simulink model "model2"  (R2025a)
settings: Solver=FixedStepAuto  StartTime=0.0  StopTime=3600  FixedStep=5  RelTol=1e-3
libraries: fuzblock x3
settings Model: Creator=boris  LastModifiedBy=boris

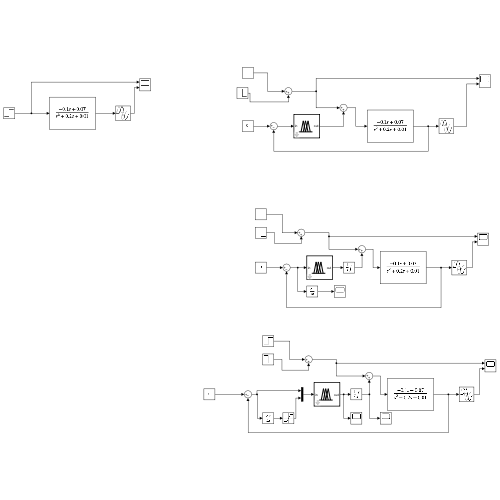
[thumbnail: Simulink's stored preview of the top-level diagram]
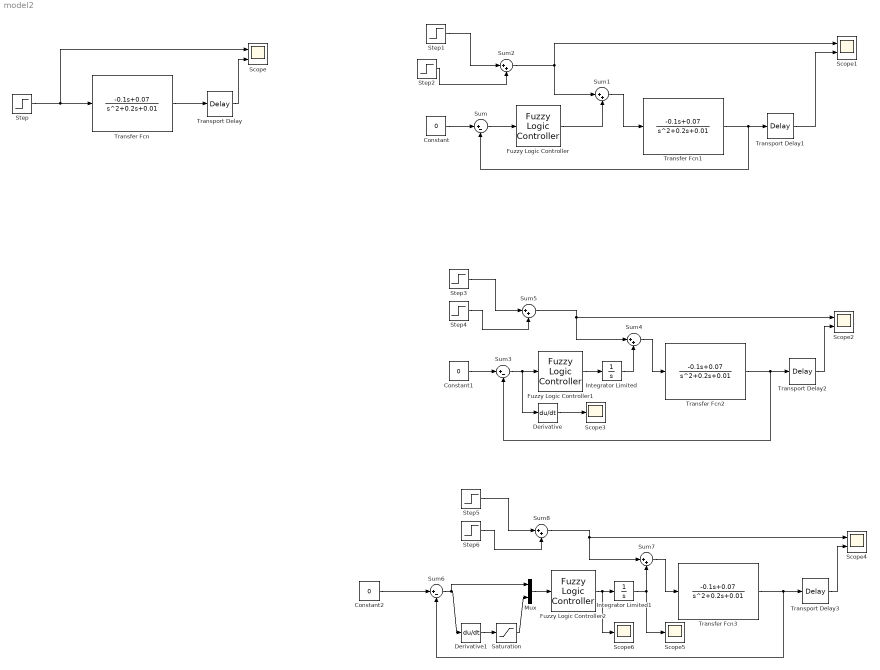
== system model2 ==
  Constant : Constant  Value=0
  Constant1 : Constant  Value=0
  Constant2 : Constant  Value=0
  Derivative : Derivative
  Derivative1 : Derivative
  Fuzzy Logic Controller : fuzblock/Fuzzy Logic  Controller  FIS='fisprvasema.fis'  OutputSampleNumber=101  DataType=double  UseLookupTable=off  NumBreakpoints=10  FuzzifiedInputs=off  RuleFiringStrengths=off  RuleOutputs=off  AggregatedOutputs=off  SimulateUsing=Interpreted execution  OutOfRangeInputValueMessage=warning  NoRuleFiredMessage=warning  EmptyOutputFuzzySetMessage=warning
  Fuzzy Logic Controller1 : fuzblock/Fuzzy Logic  Controller  FIS='fisdrugasema.fis'  OutputSampleNumber=101  DataType=double  UseLookupTable=off  NumBreakpoints=10  FuzzifiedInputs=off  RuleFiringStrengths=off  RuleOutputs=off  AggregatedOutputs=off  SimulateUsing=Interpreted execution  OutOfRangeInputValueMessage=warning  NoRuleFiredMessage=warning  EmptyOutputFuzzySetMessage=warning
  Fuzzy Logic Controller2 : fuzblock/Fuzzy Logic  Controller  FIS='fistrecasema.fis'  OutputSampleNumber=101  DataType=double  UseLookupTable=off  NumBreakpoints=10  FuzzifiedInputs=off  RuleFiringStrengths=off  RuleOutputs=off  AggregatedOutputs=off  SimulateUsing=Interpreted execution  OutOfRangeInputValueMessage=warning  NoRuleFiredMessage=warning  EmptyOutputFuzzySetMessage=warning
  Integrator Limited : Integrator  LimitOutput=on  UpperSaturationLimit=1  LowerSaturationLimit=-1
  Integrator Limited1 : Integrator  LimitOutput=on  UpperSaturationLimit=1  LowerSaturationLimit=-1
  Mux : Mux  Inputs=2
  Saturation : Saturate  UpperLimit=0.25  LowerLimit=-0.25
  Scope{,1..2,4} (4 alike) : Scope  NumInputPorts=2
      Scope settings: ActiveDisplayYMinimum=-9.2632730102427523  ActiveDisplayYMaximum=9.6776583032844812
      Scope1 settings: ActiveDisplayYMinimum=-1.7304588396468332  ActiveDisplayYMaximum=2.1411173344644125
      Scope2 settings: ActiveDisplayYMinimum=-9.7183610699907845  ActiveDisplayYMaximum=6.5365808726053523  DataLoggingVariableName=ScopeData2
      Scope4 settings: ActiveDisplayYMinimum=-14.3317272983633  ActiveDisplayYMaximum=17.948196332901027  DataLoggingVariableName=ScopeData4
  Scope3 : Scope
      settings: ActiveDisplayYMinimum=-0.796880349615698  ActiveDisplayYMaximum=0.27152824199195597  DataLoggingVariableName=ScopeData3
  Scope5 : Scope
      settings: ActiveDisplayYMinimum=-0.48698092137964122  ActiveDisplayYMaximum=1.1652201023755158  DataLoggingVariableName=ScopeData5
  Scope6 : Scope
      settings: ActiveDisplayYMinimum=-0.056817047616125514  ActiveDisplayYMaximum=0.073005722662360772  DataLoggingVariableName=ScopeData6
  Step : Step  Time=15*60  Before=-1  SampleTime=0
  Step1 : Step  Time=15*60  After=0.5  SampleTime=0
  Step2 : Step  Time=910  After=-1  SampleTime=0
  Step3 : Step  Time=15*60  After=0.5  SampleTime=0
  Step4 : Step  Time=920  After=-1  SampleTime=0
  Step5 : Step  Time=15*60  Before=0.1  After=0.5  SampleTime=0
  Step6 : Step  Time=910  After=-1  SampleTime=0
  Sum : Sum  Inputs=|+-
  Sum{1..2,4..5,7..8} (6 alike) : Sum  Inputs=|++
  Sum3 : Sum  Inputs=|+-
  Sum6 : Sum  Inputs=|+-
  Transfer Fcn{,1..3} (4 alike) : TransferFcn  Numerator=[-0.1 0.07]  Denominator=[1 0.2 0.01]
  Transport Delay{,1..3} (4 alike) : TransportDelay  DelayTime=3
  wires:
  Transfer Fcn/1 -> Transport Delay/1
  Step/1 -> Scope/1, Transfer Fcn/1
  Transfer Fcn1/1 -> Sum/2, Transport Delay1/1
  Transport Delay/1 -> Scope/2
  Constant/1 -> Sum/1
  Sum/1 -> Fuzzy Logic Controller/1
  Sum1/1 -> Transfer Fcn1/1
  Fuzzy Logic Controller/1 -> Sum1/2
  Step1/1 -> Sum2/1
  Step2/1 -> Sum2/2
  Sum2/1 -> Sum1/1, Scope1/1
  Sum5/1 -> Scope2/1, Sum4/1
  Step4/1 -> Sum5/2
  Sum3/1 -> Derivative/1, Fuzzy Logic Controller1/1
  Sum4/1 -> Transfer Fcn2/1
  Constant1/1 -> Sum3/1
  Transfer Fcn2/1 -> Sum3/2, Transport Delay2/1
  Transport Delay2/1 -> Scope2/2
  Step3/1 -> Sum5/1
  Fuzzy Logic Controller1/1 -> Integrator Limited/1
  Integrator Limited/1 -> Sum4/2
  Derivative/1 -> Scope3/1
  Step6/1 -> Sum8/2
  Sum6/1 -> Mux/1, Derivative1/1
  Transfer Fcn3/1 -> Sum6/2, Transport Delay3/1
  Constant2/1 -> Sum6/1
  Sum7/1 -> Transfer Fcn3/1
  Step5/1 -> Sum8/1
  Transport Delay3/1 -> Scope4/2
  Integrator Limited1/1 -> Scope5/1, Sum7/2
  Sum8/1 -> Scope4/1, Sum7/1
  Fuzzy Logic Controller2/1 -> Scope6/1, Integrator Limited1/1
  Derivative1/1 -> Saturation/1
  Mux/1 -> Fuzzy Logic Controller2/1
  Saturation/1 -> Mux/2
  Transport Delay1/1 -> Scope1/2
